simulink model "RecvRStEnCtrl"  (R2018b)
settings: Solver=FixedStepDiscrete  StartTime=0.0  StopTime=10.0  FixedStep=0.01  RelTol=1e-3
undefined symbols (not defined in the file or in its folder): data, PassStFtEn_Clear, PassStFtEn_Set, SecRwRtStBkReclnEn_Clear, SecRwRtStBkReclnEn_Set, SecRwRtStLgrstUpwdDnwdEn_Clear, SecRwRtStLgrstUpwdDnwdEn_Set
libraries: simulink x1
settings Model: Creator=sn2xws  LastModifiedBy=sn2xws
settings DataIOCC: SaveFormat=StructureWithTime
settings OptimizationCC: DefaultParameterBehavior=Inlined  EnhancedBackFolding=on  PassReuseOutputArgsAs=Individual arguments  ZeroExternalMemoryAtStartup=off  ZeroInternalMemoryAtStartup=off  OptimizeBlockOrder=speed  DifferentSizesBufferReuse=on  OptimizationCustomize=off
settings DebuggingCC: ParameterTunabilityLossMsg=error
settings ModelReferenceCC: ModelReferenceNumInstancesAllowed=Single
settings SFSimCC: MATLABDynamicMemAlloc=off
settings RTWCC: SystemTargetFile=autosar.tlc  GenCodeOnly=on  TemplateMakefile=ert_default_tmf  Description=AUTOSAR  GenerateReport=on  IncludeHyperlinkInReport=on  LaunchReport=on  GenerateTraceInfo=on  GenerateTraceReport=on  GenerateTraceReportSl=on  GenerateTraceReportSf=on  GenerateTraceReportEml=on
settings CodeAppCC: ForceParamTrailComments=on  IgnoreCustomStorageClasses=off  OperatorAnnotations=on  SimulinkDataObjDesc=on  SFDataObjDesc=on  InsertBlockDesc=on
settings STFCustomTargetCC: TargetLangStandard=C99 (ISO)  MultiwordLength=256  ParMdlRefBuildCompliant=on  CompOptLevelCompliant=on  IncludeMdlTerminateFcn=off  CombineOutputUpdateFcns=on  SuppressErrorStatus=on  ERTCustomFileBanners=on  SupportNonFinite=off  SupportComplex=off  SupportContinuousTime=off  SupportNonInlinedSFcns=off  RemoveResetFunc=on  MATLABClassNameForMDSCustomization=Simulink.SoftwareTarget.ERTCustomization  AutosarCompliant=on  UseToolchainInfoCompliant=on  LookupTableObjectStructAxisOrder=2,1,3,4,...  LUTObjectStructOrderEvenSpacing=Size,Table,Breakpoints  SystemTargetFile=autosar.tlc
settings ERTTargetCC: TargetLangStandard=C99 (ISO)  ConcurrentExecutionCompliant=off  IncludeMdlTerminateFcn=off  SuppressErrorStatus=on  SupportNonFinite=off  SupportComplex=off  ModelStepFunctionPrototypeControlCompliant=off  CPPClassGenCompliant=off  AutosarCompliant=on  LookupTableObjectStructAxisOrder=2,1,3,4,...  LUTObjectStructOrderEvenSpacing=Size,Table,Breakpoints  InlinedParameterPlacement=NonHierarchical  ERTCustomFileTemplate=example_file_process.tlc  ERTFilePackagingFormat=Compact

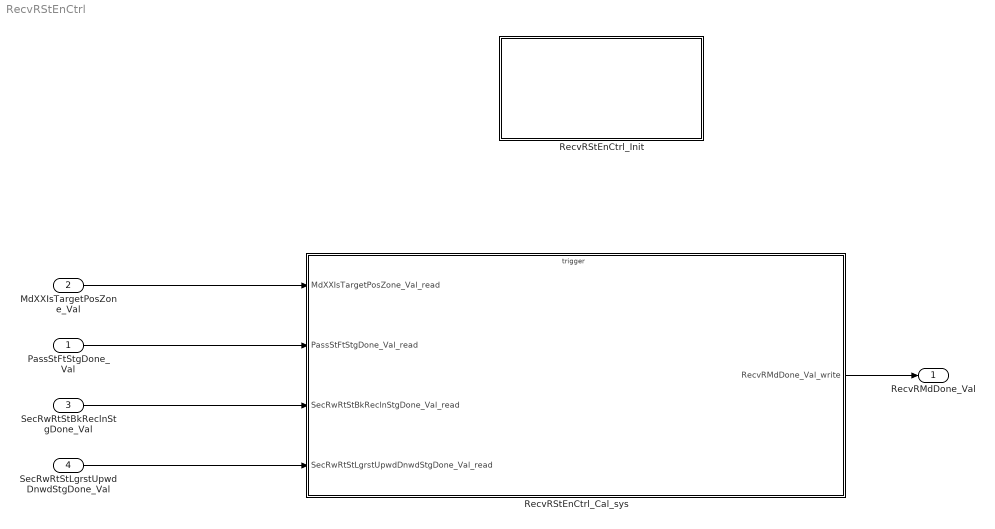
== system RecvRStEnCtrl ==
  PassStFtStgDone_Val : Inport  OutDataTypeStr=boolean  PortDimensions=1
  MdXXIsTargetPosZone_Val : Inport  Port=2  OutDataTypeStr=uint32  PortDimensions=1
  SecRwRtStBkReclnStgDone_Val : Inport  Port=3  OutDataTypeStr=boolean  PortDimensions=1
  SecRwRtStLgrstUpwdDnwdStgDone_Val : Inport  Port=4  OutDataTypeStr=boolean  PortDimensions=1
  RecvRStEnCtrl_Cal_sys : Subsystem
  RecvRStEnCtrl_Init : Subsystem
  RecvRMdDone_Val : Outport  OutDataTypeStr=uint8  PortDimensions=1
  wires:
  RecvRStEnCtrl_Cal_sys/1(RecvRMdDone_Val_write) -> RecvRMdDone_Val/1
  PassStFtStgDone_Val/1 -> RecvRStEnCtrl_Cal_sys/2(PassStFtStgDone_Val_read)
  MdXXIsTargetPosZone_Val/1 -> RecvRStEnCtrl_Cal_sys/1(MdXXIsTargetPosZone_Val_read)
  SecRwRtStBkReclnStgDone_Val/1 -> RecvRStEnCtrl_Cal_sys/3(SecRwRtStBkReclnStgDone_Val_read)
  SecRwRtStLgrstUpwdDnwdStgDone_Val/1 -> RecvRStEnCtrl_Cal_sys/4(SecRwRtStLgrstUpwdDnwdStgDone_Val_read)

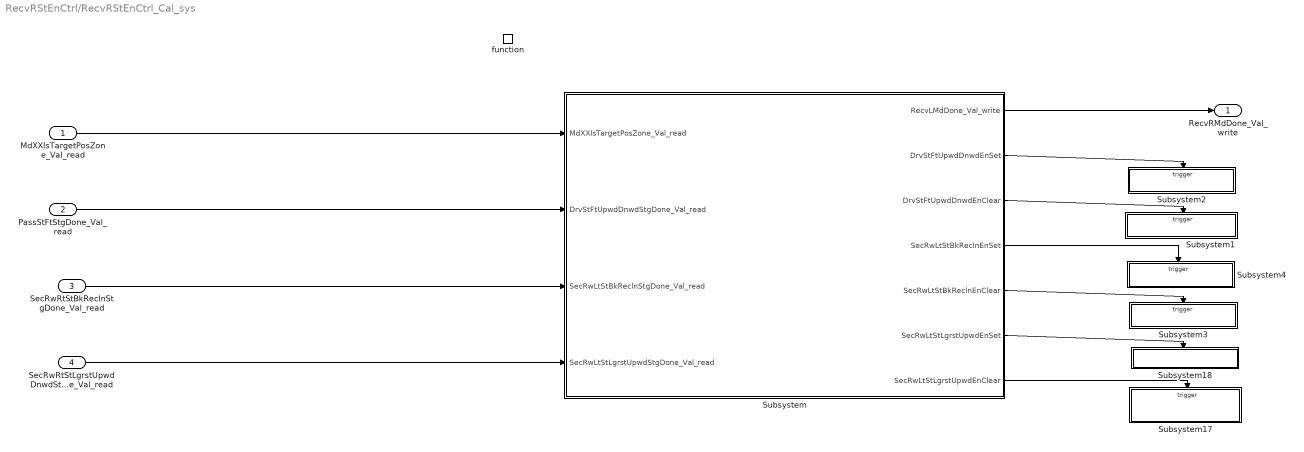
== system RecvRStEnCtrl/RecvRStEnCtrl_Cal_sys ==
  MdXXIsTargetPosZone_Val_read : Inport
  PassStFtStgDone_Val_read : Inport  Port=2
  SecRwRtStBkReclnStgDone_Val_read : Inport  Port=3
  SecRwRtStLgrstUpwdDnwdStgDone_Val_read : Inport  Port=4
  function : TriggerPort  TriggerType=function-call  IsSimulinkFunction=on  FunctionName=RecvRStEnCtrl_Cal  VariantControl=(inherit)
  Subsystem : Subsystem
  Subsystem1 : Subsystem
  Subsystem17 : Subsystem
  Subsystem18 : Subsystem
  Subsystem2 : Subsystem
  Subsystem3 : Subsystem
  Subsystem4 : Subsystem
  RecvRMdDone_Val_write : Outport
      settings: EnsureOutportIsVirtual=on
  wires:
  Subsystem/1(RecvLMdDone_Val_write) -> RecvRMdDone_Val_write/1
  MdXXIsTargetPosZone_Val_read/1 -> Subsystem/1(MdXXIsTargetPosZone_Val_read)
  PassStFtStgDone_Val_read/1 -> Subsystem/2(DrvStFtUpwdDnwdStgDone_Val_read)
  SecRwRtStBkReclnStgDone_Val_read/1 -> Subsystem/3(SecRwLtStBkReclnStgDone_Val_read)
  SecRwRtStLgrstUpwdDnwdStgDone_Val_read/1 -> Subsystem/4(SecRwLtStLgrstUpwdStgDone_Val_read)
  Subsystem/7(SecRwLtStLgrstUpwdEnClear) -> Subsystem17/Trigger
  Subsystem/6(SecRwLtStLgrstUpwdEnSet) -> Subsystem18/Trigger
  Subsystem/2(DrvStFtUpwdDnwdEnSet) -> Subsystem2/Trigger
  Subsystem/5(SecRwLtStBkReclnEnClear) -> Subsystem3/Trigger
  Subsystem/3(DrvStFtUpwdDnwdEnClear) -> Subsystem1/Trigger
  Subsystem/4(SecRwLtStBkReclnEnSet) -> Subsystem4/Trigger

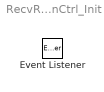
== system RecvRStEnCtrl/RecvRStEnCtrl_Init ==
  Event Listener : EventListener  EventName=reset

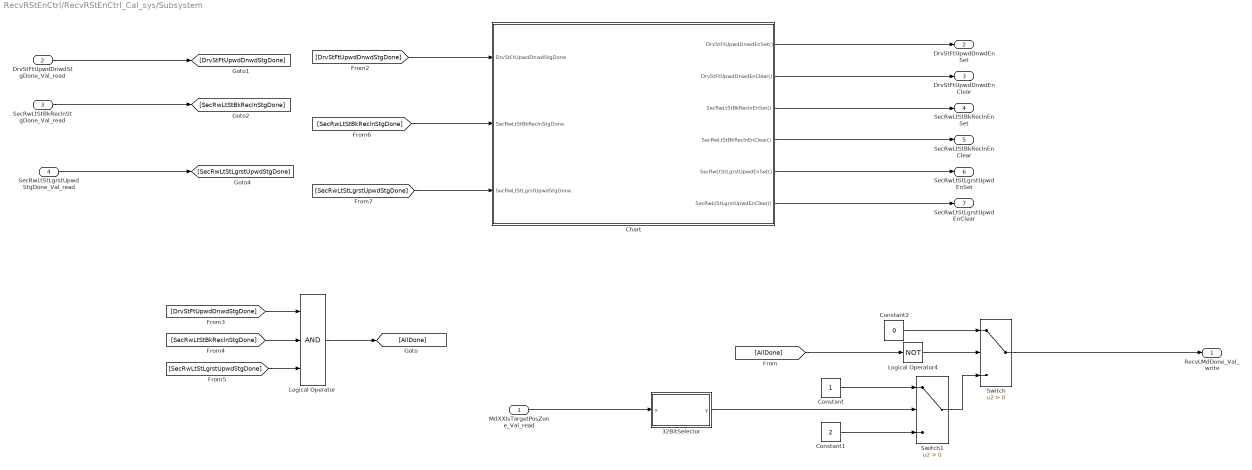
== system RecvRStEnCtrl/RecvRStEnCtrl_Cal_sys/Subsystem ==
  MdXXIsTargetPosZone_Val_read : Inport
  DrvStFtUpwdDnwdStgDone_Val_read : Inport  Port=2
  SecRwLtStBkReclnStgDone_Val_read : Inport  Port=3
  SecRwLtStLgrstUpwdStgDone_Val_read : Inport  Port=4
  32BitSelector : Subsystem  mask(32 Bit Selector){BitNum=12}
      mask prompts: BitNum "Select Bit Number"
      mask help: Allows selection of a particular bit (0-31) out of a packed word up to 32 bits long. Output will be true if the bit number selected via the mask parameter is equal to one.
      mask TypeOptions BitNum: 0 | 1 | 2 | 3 | 4 | 5 | 6 | 7 | 8 | 9 | 10 | 11 | 12 | 13 | 14 | 15 | 16 | 17 | 18 | 19 | 20 | 21 | 22 | 23 | 24 | 25 | 26 | 27 | 28 | 29 | 30 | 31
      mask Display:
      | text(0.5, 0.8,'BIT','horizontalAlignment','center')
      | text(0.5, 0.5,'SELECTOR','horizontalAlignment','center')
      | text(0.5, 0.2,['-- Bit ',char(get_param(gcb,'BitNum')),' --'],'horizontalAlignment','center')
  Chart : Stateflow chart  TreatAsAtomicUnit=on
  Constant : Constant  OutDataTypeStr=uint8
  Constant1 : Constant  Value=2  OutDataTypeStr=uint8
  Constant2 : Constant  Value=0  OutDataTypeStr=uint8
  Logical Operator : Logic  Inputs=3  AllPortsSameDT=off  OutDataTypeStr=boolean
  Logical Operator4 : Logic  Operator=NOT  AllPortsSameDT=off  OutDataTypeStr=boolean
  Switch : Switch  Criteria=u2 > Threshold
  Switch1 : Switch  Criteria=u2 > Threshold
  RecvLMdDone_Val_write : Outport
      settings: EnsureOutportIsVirtual=on
  DrvStFtUpwdDnwdEnSet : Outport  Port=2
  DrvStFtUpwdDnwdEnClear : Outport  Port=3
  SecRwLtStBkReclnEnSet : Outport  Port=4
  SecRwLtStBkReclnEnClear : Outport  Port=5
  SecRwLtStLgrstUpwdEnSet : Outport  Port=6
  SecRwLtStLgrstUpwdEnClear : Outport  Port=7
  wires:
  Switch/1 -> RecvLMdDone_Val_write/1
  MdXXIsTargetPosZone_Val_read/1 -> 32BitSelector/1(x)
  Switch1/1 -> Switch/3
  DrvStFtUpwdDnwdStgDone_Val_read/1 -> [DrvStFtUpwdDnwdStgDone]
  SecRwLtStBkReclnStgDone_Val_read/1 -> [SecRwLtStBkReclnStgDone]
  SecRwLtStLgrstUpwdStgDone_Val_read/1 -> [SecRwLtStLgrstUpwdStgDone]
  [DrvStFtUpwdDnwdStgDone] -> Logical Operator/1
  [SecRwLtStBkReclnStgDone] -> Logical Operator/2
  [SecRwLtStLgrstUpwdStgDone] -> Logical Operator/3
  Logical Operator/1 -> [AllDone]
  [DrvStFtUpwdDnwdStgDone] -> Chart/1(DrvStFtUpwdDnwdStgDone)
  [SecRwLtStBkReclnStgDone] -> Chart/2(SecRwLtStBkReclnStgDone)
  [SecRwLtStLgrstUpwdStgDone] -> Chart/3(SecRwLtStLgrstUpwdStgDone)
  Chart/1(DrvStFtUpwdDnwdEnSet()) -> DrvStFtUpwdDnwdEnSet/1
  Chart/2(DrvStFtUpwdDnwdEnClear()) -> DrvStFtUpwdDnwdEnClear/1
  Chart/3(SecRwLtStBkReclnEnSet()) -> SecRwLtStBkReclnEnSet/1
  Chart/4(SecRwLtStBkReclnEnClear()) -> SecRwLtStBkReclnEnClear/1
  Chart/5(SecRwLtStLgrstUpwdEnSet()) -> SecRwLtStLgrstUpwdEnSet/1
  Chart/6(SecRwLtStLgrstUpwdEnClear()) -> SecRwLtStLgrstUpwdEnClear/1
  Constant2/1 -> Switch/1
  Constant1/1 -> Switch1/3
  Constant/1 -> Switch1/1
  [AllDone] -> Logical Operator4/1
  Logical Operator4/1 -> Switch/2
  32BitSelector/1(y) -> Switch1/2

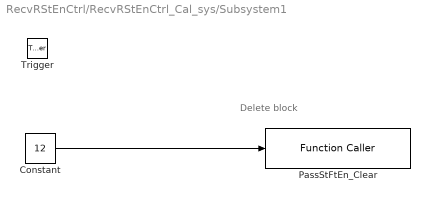
== system RecvRStEnCtrl/RecvRStEnCtrl_Cal_sys/Subsystem1 ==
  note: Delete block
  Trigger : TriggerPort  TriggerType=function-call  VariantControl=Variant  PortDimensions=1
  Constant : Constant  Value=12  OutDataTypeStr=uint8
  PassStFtEn_Clear : FunctionCaller  FunctionPrototype=PassStFtEn_Clear(data)  InputArgumentSpecifications=uint8(1)
  wires:
  Constant/1 -> PassStFtEn_Clear/1

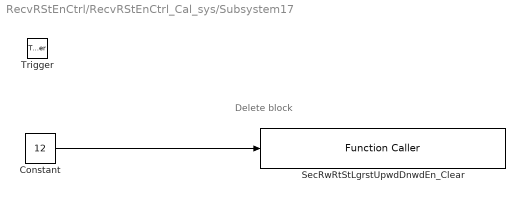
== system RecvRStEnCtrl/RecvRStEnCtrl_Cal_sys/Subsystem17 ==
  note: Delete block
  Trigger : TriggerPort  TriggerType=function-call  VariantControl=Variant  PortDimensions=1
  Constant : Constant  Value=12  OutDataTypeStr=uint8
  SecRwRtStLgrstUpwdDnwdEn_Clear : FunctionCaller  FunctionPrototype=SecRwRtStLgrstUpwdDnwdEn_Clear(data)  InputArgumentSpecifications=uint8(1)
  wires:
  Constant/1 -> SecRwRtStLgrstUpwdDnwdEn_Clear/1

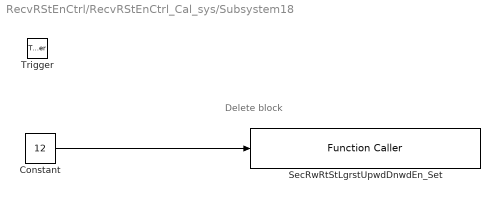
== system RecvRStEnCtrl/RecvRStEnCtrl_Cal_sys/Subsystem18 ==
  note: Delete block
  Trigger : TriggerPort  TriggerType=function-call  VariantControl=Variant  PortDimensions=1
  Constant : Constant  Value=12  OutDataTypeStr=uint8
  SecRwRtStLgrstUpwdDnwdEn_Set : FunctionCaller  FunctionPrototype=SecRwRtStLgrstUpwdDnwdEn_Set(data)  InputArgumentSpecifications=uint8(1)
  wires:
  Constant/1 -> SecRwRtStLgrstUpwdDnwdEn_Set/1

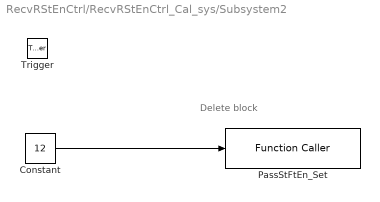
== system RecvRStEnCtrl/RecvRStEnCtrl_Cal_sys/Subsystem2 ==
  note: Delete block
  Trigger : TriggerPort  TriggerType=function-call  VariantControl=Variant  PortDimensions=1
  Constant : Constant  Value=12  OutDataTypeStr=uint8
  PassStFtEn_Set : FunctionCaller  FunctionPrototype=PassStFtEn_Set(data)  InputArgumentSpecifications=uint8(1)
  wires:
  Constant/1 -> PassStFtEn_Set/1

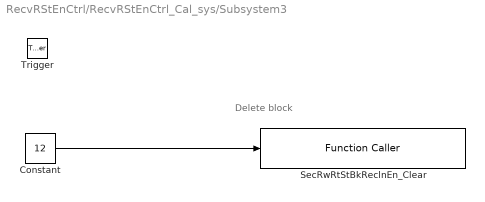
== system RecvRStEnCtrl/RecvRStEnCtrl_Cal_sys/Subsystem3 ==
  note: Delete block
  Trigger : TriggerPort  TriggerType=function-call  VariantControl=Variant  PortDimensions=1
  Constant : Constant  Value=12  OutDataTypeStr=uint8
  SecRwRtStBkReclnEn_Clear : FunctionCaller  FunctionPrototype=SecRwRtStBkReclnEn_Clear(data)  InputArgumentSpecifications=uint8(1)
  wires:
  Constant/1 -> SecRwRtStBkReclnEn_Clear/1

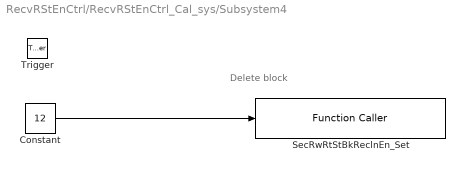
== system RecvRStEnCtrl/RecvRStEnCtrl_Cal_sys/Subsystem4 ==
  note: Delete block
  Trigger : TriggerPort  TriggerType=function-call  VariantControl=Variant  PortDimensions=1
  Constant : Constant  Value=12  OutDataTypeStr=uint8
  SecRwRtStBkReclnEn_Set : FunctionCaller  FunctionPrototype=SecRwRtStBkReclnEn_Set(data)  InputArgumentSpecifications=uint8(1)
  wires:
  Constant/1 -> SecRwRtStBkReclnEn_Set/1

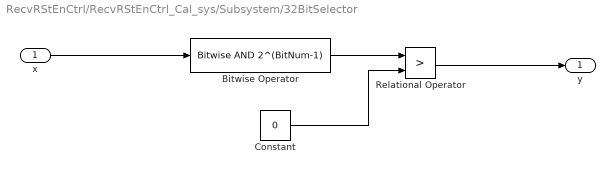
== system RecvRStEnCtrl/RecvRStEnCtrl_Cal_sys/Subsystem/32BitSelector ==
  x : Inport
  Bitwise Operator : simulink/Logic and Bit Operations/Bitwise Operator  logicop=AND  UseBitMask=on  BitMask=2^(BitNum-1)  BitMaskRealWorld=Stored Integer
  Constant : Constant  Value=0  OutDataTypeStr=uint32
  Relational Operator : RelationalOperator  Operator=>  OutDataTypeStr=boolean  RndMeth=Simplest
  y : Outport
  wires:
  Relational Operator/1 -> y/1
  Constant/1 -> Relational Operator/2
  x/1 -> Bitwise Operator/1
  Bitwise Operator/1 -> Relational Operator/1

== stateflow chart RecvRStEnCtrl/RecvRStEnCtrl_Cal_sys/Subsystem/Chart ==
  (default) -> (junction 11)
  (junction 11) -> (junction 13)
  (junction 13) -> (junction 15) [order 1] : [DrvStFtUpwdDnwdStgDone]
  (junction 13) -> (junction 19) [order 2] : {DrvStFtUpwdDnwdEnSet;}
  (junction 15) -> (junction 17) : {DrvStFtUpwdDnwdEnClear;}
  (junction 17) -> (junction 19)
  (junction 19) -> (junction 24)
  (junction 24) -> (junction 26) [order 1] : [SecRwLtStBkReclnStgDone]
  (junction 24) -> (junction 30) [order 2] : {SecRwLtStBkReclnEnSet;}
  (junction 26) -> (junction 28) : {SecRwLtStBkReclnEnClear;}
  (junction 28) -> (junction 30)
  (junction 30) -> (junction 34)
  (junction 34) -> (junction 36) [order 1] : [SecRwLtStLgrstUpwdStgDone]
  (junction 34) -> (junction 40) [order 2] : {SecRwLtStLgrstUpwdEnSet;}
  (junction 36) -> (junction 38) : {SecRwLtStLgrstUpwdEnClear;}
  (junction 38) -> (junction 40)
  data: DrvStFtUpwdDnwdStgDone input; SecRwLtStBkReclnStgDone input; SecRwLtStLgrstUpwdStgDone input
  events: DrvStFtUpwdDnwdEnSet output FUNCTION_CALL_EVENT; DrvStFtUpwdDnwdEnClear output FUNCTION_CALL_EVENT; SecRwLtStBkReclnEnSet output FUNCTION_CALL_EVENT; SecRwLtStBkReclnEnClear output FUNCTION_CALL_EVENT; SecRwLtStLgrstUpwdEnSet output FUNCTION_CALL_EVENT; SecRwLtStLgrstUpwdEnClear output FUNCTION_CALL_EVENT
